simulink model "realtsim"  (R2022b)
settings: Solver=FixedStepAuto  StartTime=0.0  StopTime=9  FixedStep=0.001  RelTol=1e-3
values from neighbouring files (symbols this model uses):
  d = 1/sqrt(2)    [parameters.m]
  K = lqr(sysG, Q, R)    [LQR_Bryson.m]    (also in LQR_design.m; stateSpace_Integral.m = K(2:end); stateSpace_Nominal.m = acker(A,B,eig); stateSpace_design.m = K(2:end))
  Ki = 0    [LQR_Bryson.m]    (also in LQR_design.m; stateSpace_Integral.m = K(1); stateSpace_Nominal.m; stateSpace_design.m = K(1))
  Nu = N(end)    [LQR_Bryson.m]    (also in stateSpace_Integral.m; stateSpace_Nominal.m; stateSpace_design.m)
  Nx = N(1:4)    [LQR_Bryson.m]    (also in stateSpace_Integral.m; stateSpace_Nominal.m; stateSpace_design.m)
  omega_c = 2*pi*50    (= 314.159265359)    [parameters.m]
  rads2rpm = 60/2/pi    (= 9.54929658551)    [parameters.m]
  rpm2rads = 2*pi/60    (= 0.10471975512)    [parameters.m]
  V2deg = 170/2.5    (= 68)    [parameters.m]
undefined symbols (not defined in the file or in its folder): DiscIntNeverNeededParam, National_Instruments, PCIe, sens
libraries: sldrtlib x3, hdlsllib x1
settings Model: SimulationMode=external  ExtModeTrigDuration=100001  ExtModeTrigDurationFloating=100001  Creator=lucas  LastModifiedBy=gottardofi
settings DataIOCC: ReturnWorkspaceOutputs=off
settings HardwareCC: ProdBitPerLong=64  ProdHWDeviceType=Intel->x86-64 (Linux 64)
settings RTWCC: Description=Simulink Desktop Real-Time  SystemTargetFile=sldrt.tlc  TemplateMakefile=sldrt.tmf  RTWCompilerOptimization=on
settings CodeAppCC: MaxIdLength=95
settings SimulinkDesktopRealTimeCC: TargetLibSuffix=_sldrt.a  TargetPreCompLibLocation=C:\Program Files\MATLAB\R2022b\toolbox\sldrt\lib\win64

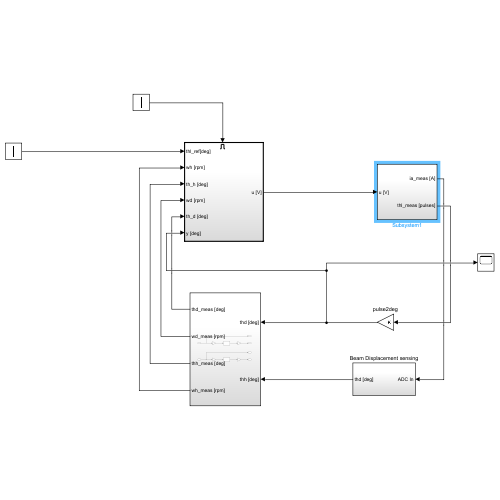
[thumbnail: Simulink's stored preview of the top-level diagram]
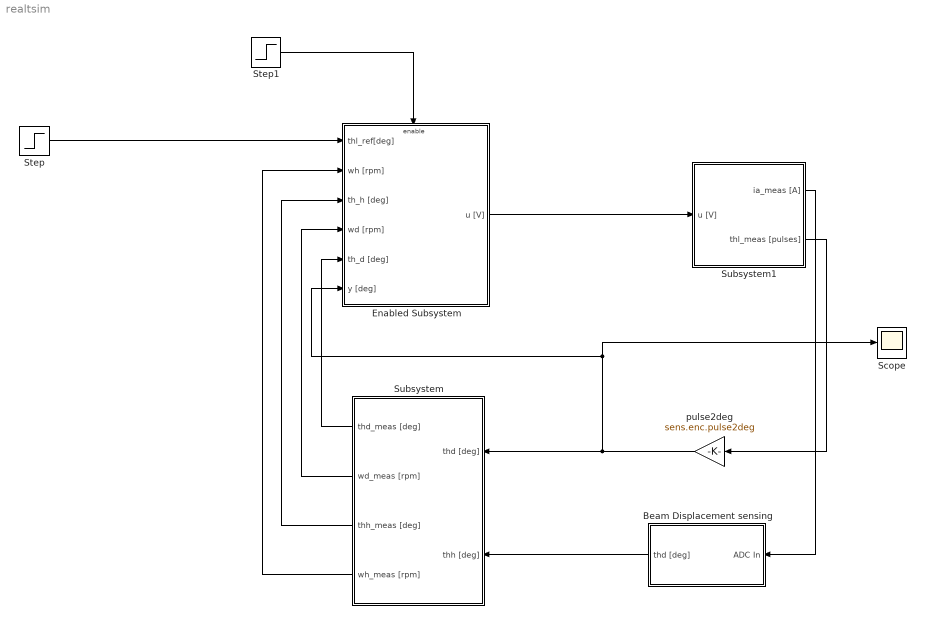
== system realtsim ==
  Beam Displacement sensing : Subsystem
  Enabled Subsystem : Subsystem  TreatAsAtomicUnit=on
  Scope : Scope
  Step : Step  After=50
  Step1 : Step  Time=0  After=50
  Subsystem : Subsystem
  Subsystem1 : Subsystem
  pulse2deg : Gain  Gain=sens.enc.pulse2deg
  wires:
  Step1/1 -> Enabled Subsystem/Enable
  Subsystem1/1(ia_meas [A]) -> Beam Displacement sensing/1(ADC In)
  Beam Displacement sensing/1(thd [deg]) -> Subsystem/2(thh [deg])
  pulse2deg/1 -> Subsystem/1(thd [deg]), Enabled Subsystem/6(y [deg]), Scope/1
  Subsystem1/2(thl_meas [pulses]) -> pulse2deg/1
  Step/1 -> Enabled Subsystem/1(thl_ref[deg])
  Subsystem/3(thh_meas [deg]) -> Enabled Subsystem/3(th_h [deg])
  Subsystem/1(thd_meas [deg]) -> Enabled Subsystem/5(th_d [deg])
  Subsystem/4(wh_meas [rpm]) -> Enabled Subsystem/2(wh [rpm])
  Subsystem/2(wd_meas [rpm]) -> Enabled Subsystem/4(wd [rpm])
  Enabled Subsystem/1(u [V]) -> Subsystem1/1(u [V])

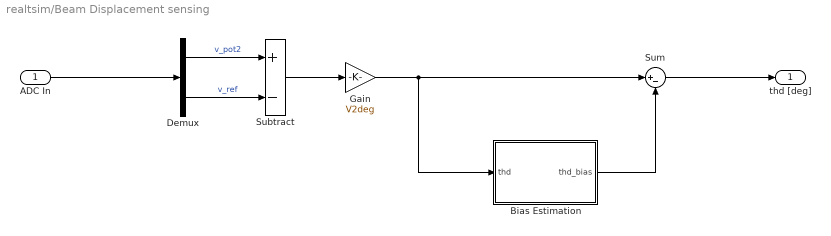
== system realtsim/Beam Displacement sensing ==
  ADC In : Inport
  Bias Estimation : Subsystem
  Demux : Demux  Outputs=2
  Gain : Gain  Gain=V2deg
  Subtract : Sum  Inputs=+-
  Sum : Sum  Inputs=|+-
  thd [deg] : Outport
  wires:
  Bias Estimation/1(thd_bias) -> Sum/2
  Sum/1 -> thd [deg]/1
  Gain/1 -> Sum/1, Bias Estimation/1(thd)
  Subtract/1 -> Gain/1
  ADC In/1 -> Demux/1
  Demux/1 -> Subtract/1  "v_pot2"
  Demux/2 -> Subtract/2  "v_ref"

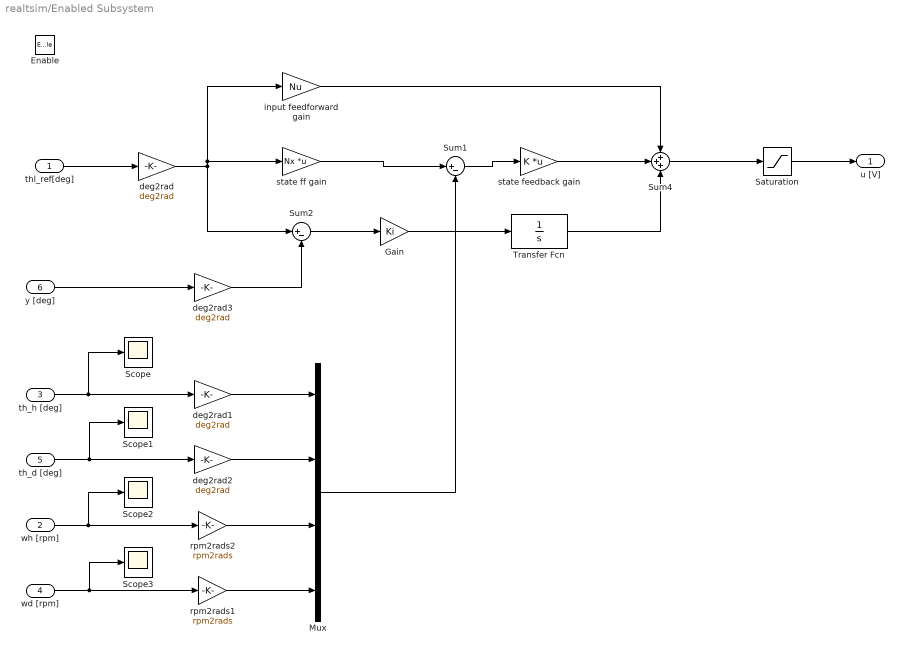
== system realtsim/Enabled Subsystem ==
  thl_ref[deg] : Inport
  wh [rpm] : Inport  Port=2
  th_h [deg] : Inport  Port=3
  wd [rpm] : Inport  Port=4
  th_d [deg] : Inport  Port=5
  y [deg] : Inport  Port=6
  Enable : EnablePort
  " Saturation" : Saturate  UpperLimit=12  LowerLimit=-12
  Gain : Gain  Gain=Ki
  Mux : Mux
  Scope{,1..3} (4 alike) : Scope
  Sum1 : Sum  Inputs=|+-
  Sum2 : Sum  Inputs=|+-
  Sum4 : Sum  Inputs=+++
  Transfer Fcn : TransferFcn  Numerator=1  Denominator=[1 0]
  deg2rad{,1..3} (4 alike) : Gain  Gain=deg2rad
  input feedforward gain : Gain  Gain=Nu
  rpm2rads1 : Gain  Gain=rpm2rads
  rpm2rads2 : Gain  Gain=rpm2rads
  state feedback gain : Gain  Gain=K  Multiplication=Matrix(K*u) (u vector)
  state ff gain : Gain  Gain=Nx  Multiplication=Matrix(K*u) (u vector)
  u [V] : Outport
  wires:
  thl_ref[deg]/1 -> deg2rad/1
  Mux/1 -> Sum1/2
  th_d [deg]/1 -> Scope1/1, deg2rad2/1
  deg2rad1/1 -> Mux/1
  wh [rpm]/1 -> Scope2/1, rpm2rads2/1
  Sum2/1 -> Gain/1
  Transfer Fcn/1 -> Sum4/3
  Gain/1 -> Transfer Fcn/1
  deg2rad3/1 -> Sum2/2
  th_h [deg]/1 -> Scope/1, deg2rad1/1
  Sum1/1 -> state feedback gain/1
  deg2rad/1 -> state ff gain/1, input feedforward gain/1, Sum2/1
  wd [rpm]/1 -> Scope3/1, rpm2rads1/1
  input feedforward gain/1 -> Sum4/1
  deg2rad2/1 -> Mux/2
  " Saturation"/1 -> u [V]/1
  y [deg]/1 -> deg2rad3/1
  rpm2rads2/1 -> Mux/3
  rpm2rads1/1 -> Mux/4
  state feedback gain/1 -> Sum4/2
  Sum4/1 -> " Saturation"/1
  state ff gain/1 -> Sum1/1

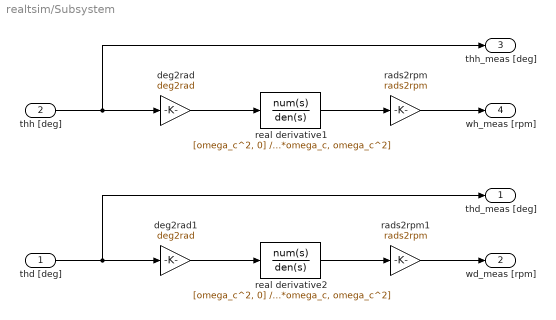
== system realtsim/Subsystem ==
  thd [deg] : Inport
  thh [deg] : Inport  Port=2
  deg2rad : Gain  Gain=deg2rad
  deg2rad1 : Gain  Gain=deg2rad
  rads2rpm : Gain  Gain=rads2rpm
  rads2rpm1 : Gain  Gain=rads2rpm
  real derivative1 : TransferFcn  Numerator=[omega_c^2, 0]  Denominator=[1, 2*d*omega_c, omega_c^2]
  real derivative2 : TransferFcn  Numerator=[omega_c^2, 0]  Denominator=[1, 2*d*omega_c, omega_c^2]
  thd_meas [deg] : Outport
  wd_meas [rpm] : Outport  Port=2
  thh_meas [deg] : Outport  Port=3
  wh_meas [rpm] : Outport  Port=4
  wires:
  deg2rad/1 -> real derivative1/1
  thh [deg]/1 -> thh_meas [deg]/1, deg2rad/1
  real derivative1/1 -> rads2rpm/1
  rads2rpm/1 -> wh_meas [rpm]/1
  rads2rpm1/1 -> wd_meas [rpm]/1
  thd [deg]/1 -> thd_meas [deg]/1, deg2rad1/1
  deg2rad1/1 -> real derivative2/1
  real derivative2/1 -> rads2rpm1/1

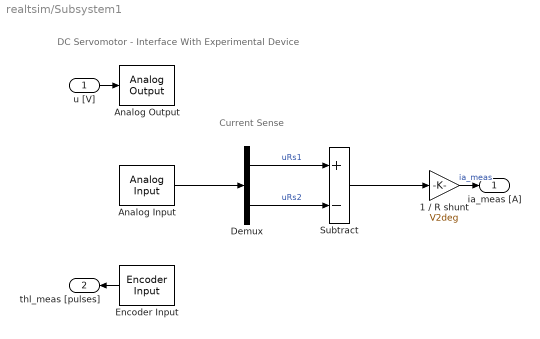
== system realtsim/Subsystem1 ==
  note: DC Servomotor - Interface With Experimental Device
  note: Current Sense
  u [V] : Inport
  1 / R shunt : Gain  Gain=V2deg
  Analog Input : sldrtlib/Analog Input  SampleTime=-1  MaxMissedTicks=10  ShowMissedTicks=off  YieldWhenWaiting=off  DrvName=National_Instruments/PCIe-6321  DrvAddress=4294967295  DrvOptions=[0 0 0 2 0 0 0]  Channels=[3,4]  RangeMode=1  VoltRange=2  DataType=1
      settings: AttributesFormatString=National Instruments\nPCIe-6321 [auto]
  Analog Output : sldrtlib/Analog Output  SampleTime=-1  MaxMissedTicks=10  ShowMissedTicks=off  YieldWhenWaiting=off  DrvName=National_Instruments/PCIe-6321  DrvAddress=4294967295  DrvOptions=[0 0 0 2 0 0 0]  Channels=1  RangeMode=1  VoltRange=1  InitialValue=0  FinalValue=0
      settings: AttributesFormatString=National Instruments\nPCIe-6321 [auto]
  Demux : Demux  Outputs=2
  Encoder Input : sldrtlib/Encoder Input  SampleTime=-1  MaxMissedTicks=10  ShowMissedTicks=off  YieldWhenWaiting=off  DrvName=National_Instruments/PCIe-6321  DrvAddress=4294967295  DrvOptions=[0 0 0 2 0 0 0]  Channels=1  QuadMode=3  IndexPulse=1  InputFilter=Inf  DataType=1
      settings: AttributesFormatString=National Instruments\nPCIe-6321 [auto]
  Subtract : Sum  Inputs=+-
  ia_meas [A] : Outport
  thl_meas [pulses] : Outport  Port=2
  wires:
  u [V]/1 -> Analog Output/1
  Subtract/1 -> 1 / R shunt/1
  Demux/2 -> Subtract/2  "uRs2"
  Encoder Input/1 -> thl_meas [pulses]/1
  1 / R shunt/1 -> ia_meas [A]/1  "ia_meas"
  Analog Input/1 -> Demux/1
  Demux/1 -> Subtract/1  "uRs1"

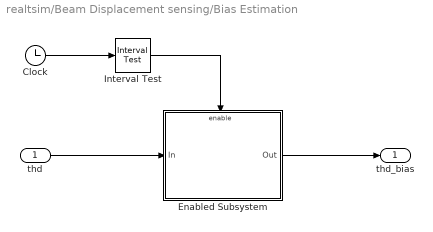
== system realtsim/Beam Displacement sensing/Bias Estimation ==
  thd : Inport
  Clock : Clock
  Enabled Subsystem : Subsystem  TreatAsAtomicUnit=on
  Interval Test : hdlsllib/Logic and Bit Operations/Interval Test  IntervalClosedRight=on  uplimit=0.5  IntervalClosedLeft=on  lowlimit=-0.5  OutDataTypeStr=boolean
  thd_bias : Outport
  wires:
  Interval Test/1 -> Enabled Subsystem/Enable
  Clock/1 -> Interval Test/1
  Enabled Subsystem/1(Out) -> thd_bias/1
  thd/1 -> Enabled Subsystem/1(In)

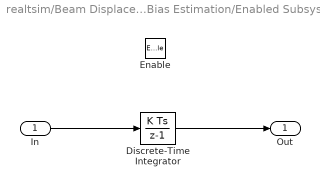
== system realtsim/Beam Displacement sensing/Bias Estimation/Enabled Subsystem ==
  In : Inport
  Enable : EnablePort
  Discrete-Time Integrator : DiscreteIntegrator  SampleTime=-1  ICPrevOutput=DiscIntNeverNeededParam  ICPrevScaledInput=DiscIntNeverNeededParam
  Out : Outport
  wires:
  Discrete-Time Integrator/1 -> Out/1
  In/1 -> Discrete-Time Integrator/1
